simulink model "blockdemo"  (Simulink 6.3)
settings: Solver=FixedStepDiscrete  StartTime=0.0  StopTime=10.0  RelTol=1e-3
InitFcn:
  | %% DSPBuilder Start
  | alt_dspbuilder_update_model(bdroot)
  | %% DSPBuilder End
libraries: allblocks_alteradspbuilder2 x11
settings Model: Creator=cpurcell  LastModifiedBy=delphick
settings DebuggingCC: MultiTaskDSMMsg=error

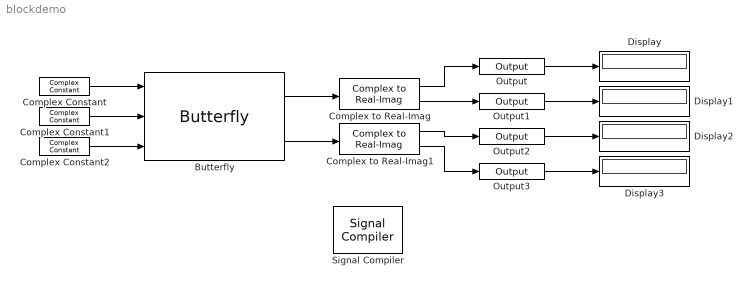
== system blockdemo ==
  Butterfly : allblocks_alteradspbuilder2/Butterfly  BusType=Signed Integer  ibwl=8  ibwr=8  pipeline=6  full_resolution=on  obwl=18  obwr=8  olsb=3  constant_W=off  W_real=1  W_imag=1  dedicated_circuitry=Auto  use_ena=off  use_aclr=off
  Complex Constant : allblocks_alteradspbuilder2/Complex Constant  mask_cst_real=5  mask_cst_imag=5  BusType=Signed Integer  bwl=8  bwr=0  SpecifyClock=off
  Complex Constant1 : allblocks_alteradspbuilder2/Complex Constant  mask_cst_real=11  mask_cst_imag=-2  BusType=Signed Integer  bwl=8  bwr=0  SpecifyClock=off
  Complex Constant2 : allblocks_alteradspbuilder2/Complex Constant  mask_cst_real=8  mask_cst_imag=8  BusType=Signed Integer  bwl=8  bwr=0  SpecifyClock=off
  Complex to Real-Imag : allblocks_alteradspbuilder2/Complex to Real-Imag  BusType=Signed Integer  bwl=18  bwr=0
  Complex to Real-Imag1 : allblocks_alteradspbuilder2/Complex to Real-Imag  BusType=Signed Integer  bwl=18  bwr=0
  Display{,1..3} (4 alike) : Display
  Output : allblocks_alteradspbuilder2/Output  iofile=C:\workspace_clean\Documentation\DesignExamples\Tutorials\UnitBlocks\Complex\Butterfly\tb_blockdemo\blockdemo_Output.capture  BusType=Inferred  bwl=8  bwr=0  PORTTYPE=Output
  Output1 : allblocks_alteradspbuilder2/Output  iofile=C:\workspace_clean\Documentation\DesignExamples\Tutorials\UnitBlocks\Complex\Butterfly\tb_blockdemo\blockdemo_Output1.capture  BusType=Inferred  bwl=8  bwr=0  PORTTYPE=Output
  Output2 : allblocks_alteradspbuilder2/Output  iofile=C:\workspace_clean\Documentation\DesignExamples\Tutorials\UnitBlocks\Complex\Butterfly\tb_blockdemo\blockdemo_Output2.capture  BusType=Inferred  bwl=8  bwr=0  PORTTYPE=Output
  Output3 : allblocks_alteradspbuilder2/Output  iofile=C:\workspace_clean\Documentation\DesignExamples\Tutorials\UnitBlocks\Complex\Butterfly\tb_blockdemo\blockdemo_Output3.capture  BusType=Inferred  bwl=8  bwr=0  PORTTYPE=Output
  Signal Compiler : allblocks_alteradspbuilder2/Signal Compiler  DeviceFamily=Stratix IV  DeviceName=AUTO  EnableSignalTap=off  SignalTapDepth=128  UseBoardBlock=off  StpUseDefaultClock=on  StpClock=clock
  wires:
  Complex Constant/1 -> Butterfly/1
  Complex Constant1/1 -> Butterfly/2
  Complex Constant2/1 -> Butterfly/3
  Butterfly/1 -> Complex to Real-Imag/1
  Butterfly/2 -> Complex to Real-Imag1/1
  Complex to Real-Imag/1 -> Output/1
  Complex to Real-Imag/2 -> Output1/1
  Complex to Real-Imag1/1 -> Output2/1
  Complex to Real-Imag1/2 -> Output3/1
  Output/1 -> Display/1
  Output1/1 -> Display1/1
  Output2/1 -> Display2/1
  Output3/1 -> Display3/1
